simulink subsystem "s2EMSSC"  (R2023b)
settings: Solver=VariableStepAuto  StartTime=0.0  StopTime=10.0  RelTol=1e-3
undefined symbols (not defined in the file): EM1, EM2, ThrmEM1, ThrmEM2
settings Model: Creator=The MathWorks, Inc.  LastModifiedBy=The MathWorks, Inc.

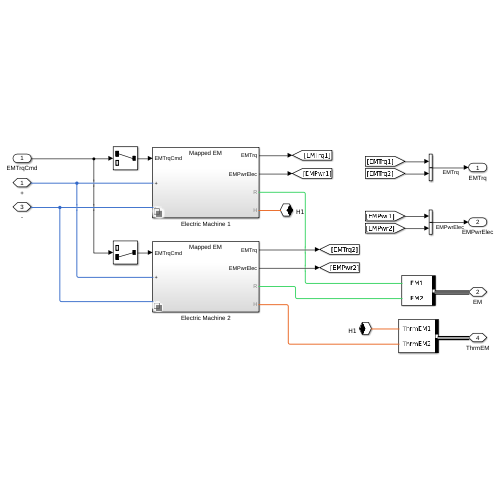
[thumbnail: Simulink's stored preview of the top-level diagram]
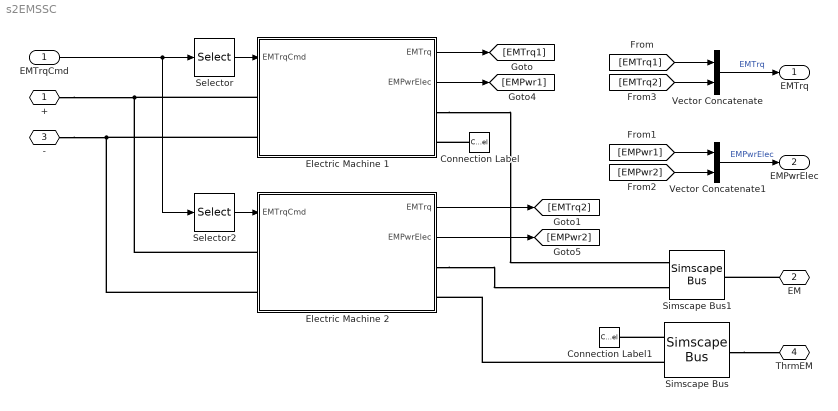
== system s2EMSSC ==
  EMTrqCmd : Inport
  Connection Label : ConnectionLabel  Label=H1
  Connection Label1 : ConnectionLabel  Label=H1
  Electric Machine 1 : Subsystem  Variant=on  VariantControlMode=label  LabelModeActiveChoice=Mapped EM
  Electric Machine 2 : Subsystem  Variant=on  VariantControlMode=label  LabelModeActiveChoice=Mapped EM
  Selector : Selector  InputPortWidth=2  IndexOptions=Index vector (dialog)  Indices=[1]  OutputSizes=1
  Selector2 : Selector  InputPortWidth=2  IndexOptions=Index vector (dialog)  Indices=[2]  OutputSizes=1
  Simscape Bus : SimscapeBus  HierarchyStrings=ThrmEM1;ThrmEM2
  Simscape Bus1 : SimscapeBus  HierarchyStrings=EM1;EM2
  Vector Concatenate : Concatenate
  Vector Concatenate1 : Concatenate
  + : PMIOPort  Side=Left
  EM : PMIOPort  Port=2  Side=Right
  - : PMIOPort  Port=3  Side=Left
  ThrmEM : PMIOPort  Port=4  Side=Right
  EMTrq : Outport
  EMPwrElec : Outport  Port=2
  wires:
  EMTrqCmd/1 -> Selector/1, Selector2/1
  Selector/1 -> Electric Machine 1/1(EMTrqCmd)
  Vector Concatenate/1 -> EMTrq/1  "EMTrq"
  Vector Concatenate1/1 -> EMPwrElec/1  "EMPwrElec"
  Selector2/1 -> Electric Machine 2/1(EMTrqCmd)
  Electric Machine 1/1(EMTrq) -> [EMTrq1]
  [EMTrq1] -> Vector Concatenate/1
  [EMTrq2] -> Vector Concatenate/2
  Electric Machine 2/1(EMTrq) -> [EMTrq2]
  Electric Machine 1/2(EMPwrElec) -> [EMPwr1]
  [EMPwr1] -> Vector Concatenate1/1
  Electric Machine 2/2(EMPwrElec) -> [EMPwr2]
  [EMPwr2] -> Vector Concatenate1/2
  connections:
  -/RConn1 -- Electric Machine 2/LConn2 -- Electric Machine 1/LConn2
  +/RConn1 -- Electric Machine 2/LConn1 -- Electric Machine 1/LConn1
  Simscape Bus/LConn2 -- Electric Machine 2/RConn2
  Simscape Bus/LConn1 -- Connection Label1/LConn1
  Connection Label/LConn1 -- Electric Machine 1/RConn2
  Simscape Bus/RConn1 -- ThrmEM/RConn1
  Electric Machine 1/RConn1 -- Simscape Bus1/LConn1
  Electric Machine 2/RConn1 -- Simscape Bus1/LConn2
  EM/RConn1 -- Simscape Bus1/RConn1

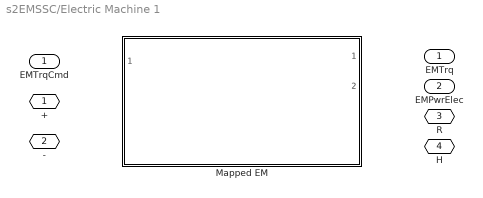
== system s2EMSSC/Electric Machine 1 ==
  EMTrqCmd : Inport
  Mapped EM : Subsystem  VariantControl=Mapped EM  ReferencedSubsystem=ElectricMachine1SSC
  + : PMIOPort  Side=Left
  - : PMIOPort  Port=2  Side=Left
  R : PMIOPort  Port=3  Side=Right
  H : PMIOPort  Port=4  Side=Right
  EMTrq : Outport  VectorParamsAs1DForOutWhenUnconnected=off
  EMPwrElec : Outport  Port=2  VectorParamsAs1DForOutWhenUnconnected=off

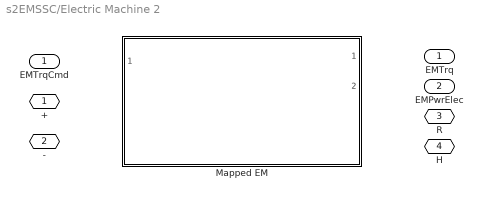
== system s2EMSSC/Electric Machine 2 ==
  EMTrqCmd : Inport
  Mapped EM : Subsystem  VariantControl=Mapped EM  ReferencedSubsystem=ElectricMachine2SSC
  + : PMIOPort  Side=Left
  - : PMIOPort  Port=2  Side=Left
  R : PMIOPort  Port=3  Side=Right
  H : PMIOPort  Port=4  Side=Right
  EMTrq : Outport  VectorParamsAs1DForOutWhenUnconnected=off
  EMPwrElec : Outport  Port=2  VectorParamsAs1DForOutWhenUnconnected=off
